simulink model "state_space_all_reduce_uio"  (R2018a)
settings: Solver=FixedStepAuto  StartTime=0.0  StopTime=3  FixedStep=tm  MaxStep=1e-4  RelTol=1e-5  AbsTol=1e-5
InitFcn:
  | SimulinkInit_linea_transmision
values from neighbouring files (symbols this model uses):
  b = 4.91    [SimulinkInit_linea_transmision.m]
  C = 1    [SimulinkInit_linea_transmision.m]
  C1 = 22e-6    (= 2.2e-05)    [SimulinkInit_linea_transmision.m]
  C2 = 22e-6    (= 2.2e-05)    [SimulinkInit_linea_transmision.m]
  C3 = 610e-6    (= 0.00061)    [SimulinkInit_linea_transmision.m]
  Cl = 20000e-6    (= 0.02)    [SimulinkInit_linea_transmision.m]
  Jd = 0.3    [SimulinkInit_linea_transmision.m]
  K = 25    [SimulinkInit_linea_transmision.m]    (also in uio_linear.m = K1+E*H)
  K1 = 9.66    [SimulinkInit_linea_transmision.m]    (also in uio_linear.m = K1')
  K11 = 0.8    [SimulinkInit_linea_transmision.m]
  K1d = 1.15    [SimulinkInit_linea_transmision.m]
  K2 = 6.97    [SimulinkInit_linea_transmision.m]
  K22 = 0.2    [SimulinkInit_linea_transmision.m]
  K2d = 1    [SimulinkInit_linea_transmision.m]
  K3 = 31.8    [SimulinkInit_linea_transmision.m]
  K33 = 0.23    [SimulinkInit_linea_transmision.m]
  K3d = 1    [SimulinkInit_linea_transmision.m]
  K4 = 15.1    [SimulinkInit_linea_transmision.m]
  Kd = 0.02    [SimulinkInit_linea_transmision.m]
  Kdc = 0.02    [SimulinkInit_linea_transmision.m]
  Kf = 1    [SimulinkInit_linea_transmision.m]
  Kh = 1.2    [SimulinkInit_linea_transmision.m]
  Ks = 21.5    [SimulinkInit_linea_transmision.m]
  Ksc = 3    [SimulinkInit_linea_transmision.m]
  Kv = 1    [SimulinkInit_linea_transmision.m]
  L = 5.2    [SimulinkInit_linea_transmision.m]
  L1 = 40e-3    (= 0.04)    [SimulinkInit_linea_transmision.m]
  L2 = 30e-3    (= 0.03)    [SimulinkInit_linea_transmision.m]
  L3 = 5e-3    (= 0.005)    [SimulinkInit_linea_transmision.m]
  L4 = 35e-6    (= 3.5e-05)    [SimulinkInit_linea_transmision.m]
  L5 = 22e-6    (= 2.2e-05)    [SimulinkInit_linea_transmision.m]
  L6 = 10e-6    (= 1e-05)    [SimulinkInit_linea_transmision.m]
  Pd = 0.1    [SimulinkInit_linea_transmision.m]
  R = 10    [SimulinkInit_linea_transmision.m]
  R1 = 0.1    [SimulinkInit_linea_transmision.m]
  R2 = 0.2    [SimulinkInit_linea_transmision.m]
  R3 = 1e-3    (= 0.001)    [SimulinkInit_linea_transmision.m]
  R4 = 0.005    [SimulinkInit_linea_transmision.m]
  R5 = 0.0012    [SimulinkInit_linea_transmision.m]
  R6 = 0.001    [SimulinkInit_linea_transmision.m]
  RL = 10    [SimulinkInit_linea_transmision.m]
  Sbin = 13.8    [SimulinkInit_linea_transmision.m]
  Svin = 2.91    [SimulinkInit_linea_transmision.m]
  T1 = 0.4    [SimulinkInit_linea_transmision.m]
  T2 = 1    [SimulinkInit_linea_transmision.m]
  T3 = 15    [SimulinkInit_linea_transmision.m]
  T4 = 2.5    [SimulinkInit_linea_transmision.m]
  Tao1d = 0.5    [SimulinkInit_linea_transmision.m]
  Tao2d = 0.125    [SimulinkInit_linea_transmision.m]
  Tcd = 0.2    [SimulinkInit_linea_transmision.m]
  Tcr = 0.01    [SimulinkInit_linea_transmision.m]
  Tf = 0.04    [SimulinkInit_linea_transmision.m]
  Tr = 950    [SimulinkInit_linea_transmision.m]
  Tt = 450    [SimulinkInit_linea_transmision.m]
  Ttd = 0.04    [SimulinkInit_linea_transmision.m]
  Tv = 0.05    [SimulinkInit_linea_transmision.m]
  V = 20    [SimulinkInit_linea_transmision.m]
  wref = 70000    [SimulinkInit_linea_transmision.m]
  X_acid = 1.2    [SimulinkInit_linea_transmision.m]
  X_meth = 0.35    [SimulinkInit_linea_transmision.m]
  Z = 3    [SimulinkInit_linea_transmision.m]
undefined symbols (not defined in the file or in its folder): Ad, ataque, Bd, c11, c12, c13, c14, C1o, c21, c22, c23, c24, C2o, c31, c32, c33, c34, C3o, c41, c42, c43, c44, C4o, Cd, F1, F2, F3, F4, H1, H2, H3, H4, K1U, K2U, K3U, K4U, T1s, T2s, T3s, T4s, T5s, tao1, tao2, taod, tm, uio1r, uio2r, uio3r, uio4r
libraries: neural x277, dsparch4 x4, powerlib_meascontrol x4, mpclib x1, simulink x1
(part 13 of 16)

== system state_space_all_reduce_uio/Function Fitting Neural Network3/Layer 2/Delays 1 ==
  "p{2}" : Inport  PortDimensions=30  SampleTime=4e-05
      mask Display: e = 0.06;c1 = [120 230 180]/255;c2 = ([120 230 180]+0)/(256+128);c3 = ([120 230 180]+128)/(256+128);patch([0 1 1 0],[0 0 1 1],c1);patch([0 1 1 1-e 1-e 0+e],[0 0 1 1-e 0+e 0+e],c2);patch([0 0 1 1-e 0+e 0+e],[0 1 1 1-e 1-e 0+e],c3);plot([0 1 1 0 0],[0 0 1 1 0]);
  mux : Mux  Inputs=1
      mask Display: e = 0.06;c1 = [120 150 230]/255;c2 = ([120 150 230]+0)/383;c3 = ([120 150 230]+128)/383;patch([0 1 1 0],[0 0 1 1],c1);patch([0 1 1 1-e 1-e 0+e],[0 0 1 1-e 0+e 0+e],c2);patch([0 0 1 1-e 0+e 0+e],[0 1 1 1-e 1-e 0+e],c3);plot([0 1 1 0 0],[0 0 1 1 0]);disp('Mux')
  "pd{2,1}" : Outport
      mask Display: e = 0.06;c1 = [120 230 180]/255;c2 = ([120 230 180]+0)/(256+128);c3 = ([120 230 180]+128)/(256+128);patch([0 1 1 0],[0 0 1 1],c1);patch([0 1 1 1-e 1-e 0+e],[0 0 1 1-e 0+e 0+e],c2);patch([0 0 1 1-e 0+e 0+e],[0 1 1 1-e 1-e 0+e],c3);plot([0 1 1 0 0],[0 0 1 1 0]);
  wires:
  "p{2}"/1 -> mux/1
  mux/1 -> "pd{2,1}"/1

== system state_space_all_reduce_uio/Function Fitting Neural Network3/Layer 2/LW{2,1} ==
  "ad{2,1}" : Inport  PortDimensions=30  SampleTime=4e-05
      mask Display: e = 0.06;c1 = [120 230 180]/255;c2 = ([120 230 180]+0)/(256+128);c3 = ([120 230 180]+128)/(256+128);patch([0 1 1 0],[0 0 1 1],c1);patch([0 1 1 1-e 1-e 0+e],[0 0 1 1-e 0+e 0+e],c2);patch([0 0 1 1-e 0+e 0+e],[0 1 1 1-e 1-e 0+e],c3);plot([0 1 1 0 0],[0 0 1 1 0]);
  "IW{2,1}(1,:)'" : Constant  Value=[-0.6108993563619720124080458845128305256366729736328125;-0.12377232021656990601510273108942783437669277191162109375;0.1986228164965912201811448767330148257315158843994140625;-0.2986234053889535999815052491612732410430908203125;-0.499479986781841578391549774096347391605377197265625;0.4244651480066325976991947754868306219577789306640625;-0.56892590557261402128830241053947247564792633056640625;-0.008160168266792812430399095546817989088594913482666015625;-0.03471042600284690582412849835236556828022003173828125;0.1662913602541268021095532958497642539441585540771484375;-0.51339807969661965802998793151346035301685333251953125;-0.11035191841669016177274187384682591073215007781982421875;0.1065034098801362905106770995189435780048370361328125;-0.387752517916231997929799035773612558841705322265625;0.25666787341159469360007960858638398349285125732421875;0.31597885591342012023829965983168222010135650634765625;-0.0106467373515204653811050405920468620024621486663818359375;-0.277670620246377064521681177211576141417026519775390625;0.024228256254273113079467094621577416546642780303955078125;0.019751607031808678105466725583028164692223072052001953125;-0.2018324091793771979386207249262952245771884918212890625;0.2218729906426324394175253473804332315921783447265625;0.3252039273491564852491819692659191787242889404296875;-0.274281505206600051405274598437245003879070281982421875;-0.149986905934014702612699920791783370077610015869140625;-0.229671358200306652275202168311807326972484588623046875;0.04070518967057305814716272607256541959941387176513671875;0.111095475677139010617366920996573753654956817626953125;-0.1194110113288310015544624320682487450540065765380859375;-0.00788339909671024151316398587141520692966878414154052734375]
      mask Display: e = 0.06;c1 = [120 150 230]/255;c2 = ([120 150 230]+0)/383;c3 = ([120 150 230]+128)/383;patch([0 1 1 0],[0 0 1 1],c1);patch([0 1 1 1-e 1-e 0+e],[0 0 1 1-e 0+e 0+e],c2);patch([0 0 1 1-e 0+e 0+e],[0 1 1 1-e 1-e 0+e],c3);plot([0 1 1 0 0],[0 0 1 1 0]);disp('weights');
  "IW{2,1}(10,:)'" : Constant  Value=[0.29635779515491955660166922825737856328487396240234375;0.2034166761778584409103842745025758631527423858642578125;-0.0023683642057664463891064610123748934711329638957977294921875;0.22124729721162073037277195908245630562305450439453125;0.3369155378131185596402019655215553939342498779296875;0.1500263956989058289348548669295269064605236053466796875;-0.2497175765352100118565914499413338489830493927001953125;-0.10301693128462863224825696306652389466762542724609375;-0.01099510239059186579579918685567463398911058902740478515625;0.115527621161523430526330002976465038955211639404296875;0.0692645313952721386474564724267111159861087799072265625;0.0119651086510804242901695459977418067865073680877685546875;0.290075191506396434792947047753841616213321685791015625;0.2032135105828389021187518892475054599344730377197265625;-0.0211155493846143203773291219249585992656648159027099609375;0.1060308181848053921125796250635175965726375579833984375;-0.1181015704355025397465084324721829034388065338134765625;0.45860412450985454935192819903022609651088714599609375;-0.20160056133213621887279032307560555636882781982421875;-0.1021768772968167648951265391588094644248485565185546875;-0.463237381515118007424547386108315549790859222412109375;-0.09568885509427126068171531869666068814694881439208984375;0.052744303583831746162768894237160566262900829315185546875;0.0475424460660857917115862392165581695735454559326171875;-0.0035101213614650308113274146393223418272100389003753662109375;-0.25541990716382245718563126501976512372493743896484375;0.528868712182579248093361456994898617267608642578125;-0.295106782712837356630330987172783352434635162353515625;-0.082279435194425432076315019003232009708881378173828125;0.07298068872108949556309909212359343655407428741455078125]
      mask Display: e = 0.06;c1 = [120 150 230]/255;c2 = ([120 150 230]+0)/383;c3 = ([120 150 230]+128)/383;patch([0 1 1 0],[0 0 1 1],c1);patch([0 1 1 1-e 1-e 0+e],[0 0 1 1-e 0+e 0+e],c2);patch([0 0 1 1-e 0+e 0+e],[0 1 1 1-e 1-e 0+e],c3);plot([0 1 1 0 0],[0 0 1 1 0]);disp('weights');
  "IW{2,1}(2,:)'" : Constant  Value=[0.09708916544488814526214781608359771780669689178466796875;0.2255772120654304380149568487468059174716472625732421875;0.003702961884490557457894066573089730809442698955535888671875;0.029624972225403896353146393494171206839382648468017578125;-0.1954796502596932439299592942916206084191799163818359375;-0.59940544466154144220837451939587481319904327392578125;0.260557299906677253265030458351247943937778472900390625;-0.63305372508061619196695346545311622321605682373046875;-0.295649046001520476867341358229168690741062164306640625;0.04053401399485075107254061776984599418938159942626953125;-0.046834290540188054652315230441672611050307750701904296875;0.08317365441290917871253185467139701358973979949951171875;0.17331529140582990766716875441488809883594512939453125;0.0275578103417470389457921697839992702938616275787353515625;0.2018023672489276665320545589565881527960300445556640625;0.06743810023460482250268199777565314434468746185302734375;-0.180275428148382765858315224249963648617267608642578125;-0.2579369278587984037898195310845039784908294677734375;-0.0921851184035180903908468508234363980591297149658203125;0.061569880123684785078186365581132122315466403961181640625;0.314599908239820258426533428064431063830852508544921875;-0.0131290228955344666361693128919796436093747615814208984375;0.033185419198564942988571857540591736324131488800048828125;-0.00933833744509623801810516141586049343459308147430419921875;-0.1033221182311379326979050574664142914116382598876953125;-0.1921781391607385869324531313395709730684757232666015625;0.055416200609459266568368462912985705770552158355712890625;-0.1488744040050123673690762871046899817883968353271484375;0.2094008490666214028497194021838367916643619537353515625;0.046990537131259495218227328905413742177188396453857421875]
      mask Display: e = 0.06;c1 = [120 150 230]/255;c2 = ([120 150 230]+0)/383;c3 = ([120 150 230]+128)/383;patch([0 1 1 0],[0 0 1 1],c1);patch([0 1 1 1-e 1-e 0+e],[0 0 1 1-e 0+e 0+e],c2);patch([0 0 1 1-e 0+e 0+e],[0 1 1 1-e 1-e 0+e],c3);plot([0 1 1 0 0],[0 0 1 1 0]);disp('weights');
  "IW{2,1}(3,:)'" : Constant  Value=[0.12460931784415903156304494814321515150368213653564453125;-0.35778269794602979292363897911855019629001617431640625;0.023278058036042138800869594206233159638941287994384765625;-0.268905202381384544896292254634317941963672637939453125;0.2125526564810290286455796149311936460435390472412109375;-0.332587259490805531303436737289302982389926910400390625;-0.1870172122518136970104052352326107211410999298095703125;-0.294072954416423726353713163916836492717266082763671875;0.0670400945985989149544792553570005111396312713623046875;0.0215328682295782801447980858711161999963223934173583984375;0.00893792162565088151027214991017899592407047748565673828125;-0.09649036626923256088073088676537736319005489349365234375;0.052689337275451102182710627630513045005500316619873046875;-0.21281430046342431072758927257382310926914215087890625;0.0208968278071027489806166244079577154479920864105224609375;0.0667961657798825658716168618411757051944732666015625;-0.00069132157059649773471476930097878721426241099834442138671875;-0.050070962703474962418592753010671003721654415130615234375;-0.08289314228870196810117221275504562072455883026123046875;0.037986939224426252703636919250129722058773040771484375;0.181202224291058422434019803404225967824459075927734375;0.274506776572543020886740805508452467620372772216796875;0.02977815686653696725105788800647133029997348785400390625;0.2139927463900734572188611082310671918094158172607421875;-0.162725233885205933237472208929830230772495269775390625;-0.019048537270349642780420396093177259899675846099853515625;0.0786097109228997836805064025611500255763530731201171875;-0.205967836298671047590147509254165925085544586181640625;0.479129205120557177810525217864778824150562286376953125;-0.2132697439127679006620752488743164576590061187744140625]
      mask Display: e = 0.06;c1 = [120 150 230]/255;c2 = ([120 150 230]+0)/383;c3 = ([120 150 230]+128)/383;patch([0 1 1 0],[0 0 1 1],c1);patch([0 1 1 1-e 1-e 0+e],[0 0 1 1-e 0+e 0+e],c2);patch([0 0 1 1-e 0+e 0+e],[0 1 1 1-e 1-e 0+e],c3);plot([0 1 1 0 0],[0 0 1 1 0]);disp('weights');
  "IW{2,1}(4,:)'" : Constant  Value=[-0.19633352528214498278202881920151412487030029296875;-0.121800271312692609537720045409514568746089935302734375;-0.0182132757588536510484633623718764283694326877593994140625;0.04471817409413435251419599580913200043141841888427734375;-0.0108854916126952215582601724008782184682786464691162109375;0.1332237321224387371909614330434123985469341278076171875;-0.146363427813941460176039299767580814659595489501953125;-0.0711709499843555526421567947181756608188152313232421875;0.25548925411243594840726700567756779491901397705078125;-0.059906029830572193883853060469846241176128387451171875;-0.1773225990205870850058289533990318886935710906982421875;-0.128281540302648655593742432756698690354824066162109375;0.039306928108965459578438839116643066518008708953857421875;-0.1122515827125971643596358262584544718265533447265625;-0.221202886936299247810921997370314784348011016845703125;0.006098252527073856101014204256216544308699667453765869140625;0.1596102041277631389259994421081501059234142303466796875;-0.1825895981040427107355839098090655170381069183349609375;0.11478182843430244364224535047469544224441051483154296875;0.0232732308372753417258227415231885970570147037506103515625;-0.3765874921128109509282921862904913723468780517578125;-0.0699864919821701347846243379535735584795475006103515625;-0.00106709298812400553251034107660188965382985770702362060546875;0.160946111283145787407278248792863450944423675537109375;0.153627959179783724064094485584064386785030364990234375;-0.01129040371139962591062744223791014519520103931427001953125;-0.1923537583599702893710770013058208860456943511962890625;-0.146999298339756057085736529188579879701137542724609375;-0.459863329862106595680160125994007103145122528076171875;-0.1125495018655740253610275658502359874546527862548828125]
      mask Display: e = 0.06;c1 = [120 150 230]/255;c2 = ([120 150 230]+0)/383;c3 = ([120 150 230]+128)/383;patch([0 1 1 0],[0 0 1 1],c1);patch([0 1 1 1-e 1-e 0+e],[0 0 1 1-e 0+e 0+e],c2);patch([0 0 1 1-e 0+e 0+e],[0 1 1 1-e 1-e 0+e],c3);plot([0 1 1 0 0],[0 0 1 1 0]);disp('weights');
  "IW{2,1}(5,:)'" : Constant  Value=[-0.341502604101319884311038777013891376554965972900390625;0.038566451327512678293185643951801466755568981170654296875;-0.1395052210143926940677516768118948675692081451416015625;0.10063509544883060542463937281354446895420551300048828125;0.1815214851574560028790727983505348674952983856201171875;-0.434218928709956430989080899962573312222957611083984375;0.408667171366868309245745649604941718280315399169921875;0.385137624400757994092003855257644318044185638427734375;-0.35508535953012343444612497478374280035495758056640625;0.395894896479553282109264955579419620335102081298828125;-0.441418591976789453923402106738649308681488037109375;0.468883832187682703107611814630217850208282470703125;0.452535260372043612875359031022526323795318603515625;-0.435690587373383897418221977204666472971439361572265625;-0.14185885407803755509092979991692118346691131591796875;0.272747534495510091101522220924380235373973846435546875;0.04098815291252873305172244045024854131042957305908203125;-0.3307976810063457673294351479853503406047821044921875;0.2101715684222978108852686318641644902527332305908203125;-0.1539716328844354109595116142372717149555683135986328125;-0.272987765307725449570597220372292213141918182373046875;0.305095574115205658838334557003690861165523529052734375;-0.04287979135288509657808475594720221124589443206787109375;-0.41147834133321092853208256201469339430332183837890625;0.53712368878818439466016343430965207517147064208984375;0.416191517197288474161354088209918700158596038818359375;0.04749985538923630346008764036014326848089694976806640625;-0.1798369007383437689906457990218768827617168426513671875;0.01525251243919280297323126660558045841753482818603515625;-0.54013565597617951841158401293796487152576446533203125]
      mask Display: e = 0.06;c1 = [120 150 230]/255;c2 = ([120 150 230]+0)/383;c3 = ([120 150 230]+128)/383;patch([0 1 1 0],[0 0 1 1],c1);patch([0 1 1 1-e 1-e 0+e],[0 0 1 1-e 0+e 0+e],c2);patch([0 0 1 1-e 0+e 0+e],[0 1 1 1-e 1-e 0+e],c3);plot([0 1 1 0 0],[0 0 1 1 0]);disp('weights');
  "IW{2,1}(6,:)'" : Constant  Value=[0.49925490638036185142567546790814958512783050537109375;0.12402283349013844271357953630285919643938541412353515625;0.07420110878195196324469407045398838818073272705078125;-0.268528915716013505399217820013291202485561370849609375;0.462956992662289235074268844982725568115711212158203125;-0.007515270830356904872837642272997982217930257320404052734375;-0.481571654503173796069148693277384154498577117919921875;-0.08387177086194898267823560900069423951208591461181640625;-0.52940697956280036162723945381003431975841522216796875;0.323217987371589021705631239456124603748321533203125;0.1568066838196668921767695792368613183498382568359375;0.40583622791357065739958898120676167309284210205078125;0.08930773221745569312446377807646058499813079833984375;-0.3258180832558463801973402951261959969997406005859375;0.1402346353061940387174644229162367992103099822998046875;-0.202497063814745581478149460963322781026363372802734375;-0.030890754278159980594775646522975875996053218841552734375;0.1144440458135578264631249112426303327083587646484375;-0.52332038790228008195981601602397859096527099609375;0.0205082634168946252584131428875480196438729763031005859375;-0.140059324007881846885226195809082128107547760009765625;0.0227385631742271603072946817292177001945674419403076171875;0.04104951059130988733070211083031608723104000091552734375;-0.44803892833890424096665583419962786138057708740234375;-0.455430901449709046868719042322481982409954071044921875;0.34017445856057137998362804864882491528987884521484375;-0.52777334503266215559591501005343161523342132568359375;0.61711177965770447340076998443691991269588470458984375;-0.1172188000697740317690431766095571219921112060546875;0.049266357298894093708074848336764262057840824127197265625]
      mask Display: e = 0.06;c1 = [120 150 230]/255;c2 = ([120 150 230]+0)/383;c3 = ([120 150 230]+128)/383;patch([0 1 1 0],[0 0 1 1],c1);patch([0 1 1 1-e 1-e 0+e],[0 0 1 1-e 0+e 0+e],c2);patch([0 0 1 1-e 0+e 0+e],[0 1 1 1-e 1-e 0+e],c3);plot([0 1 1 0 0],[0 0 1 1 0]);disp('weights');
  "IW{2,1}(7,:)'" : Constant  Value=[0.036708599756844435824110206567638670094311237335205078125;0.1096854095616091318010631994184223003685474395751953125;-0.022078643810732691277198824764127493835985660552978515625;0.61378380423222866912880135714658536016941070556640625;0.21004296218785778460613755669328384101390838623046875;-0.51994852170594063611730462071136571466922760009765625;-0.57842560919090224569316660563345067203044891357421875;0.097160600096388438640104823207366280257701873779296875;-0.37978985583719782059830549769685603678226470947265625;-0.07765784517062475356130590853354078717529773712158203125;-0.20417782875814849408158124788315035402774810791015625;-0.1448559489658842458492671312342281453311443328857421875;-0.1997818239064153844619653455083607695996761322021484375;-0.50620673707847718691965610560146160423755645751953125;-0.2243158369550604935849236198919243179261684417724609375;-0.06966453684462425854917455581016838550567626953125;0.299991235207171025312078427305095829069614410400390625;-0.1099435947310898609163842820635181851685047149658203125;0.1624020068420821971688638996056397445499897003173828125;-0.054784390240681206385442436612720484845340251922607421875;0.43531344416034845057339452978339977562427520751953125;0.2052756780230019229005478109684190712869167327880859375;-0.049654717239222601055104178158217109739780426025390625;0.07186210672408070709860083979947376064956188201904296875;0.429542962623020441181864725876948796212673187255859375;0.1707548603417280153049517821273184381425380706787109375;-0.46502172346302972361087313402094878256320953369140625;0.064153631383797760090459405546425841748714447021484375;-0.20833364336469906152871089943801052868366241455078125;-0.1460654280552280692706546005865675397217273712158203125]
      mask Display: e = 0.06;c1 = [120 150 230]/255;c2 = ([120 150 230]+0)/383;c3 = ([120 150 230]+128)/383;patch([0 1 1 0],[0 0 1 1],c1);patch([0 1 1 1-e 1-e 0+e],[0 0 1 1-e 0+e 0+e],c2);patch([0 0 1 1-e 0+e 0+e],[0 1 1 1-e 1-e 0+e],c3);plot([0 1 1 0 0],[0 0 1 1 0]);disp('weights');
  "IW{2,1}(8,:)'" : Constant  Value=[0.36685370791122784428495151587412692606449127197265625;-0.0395954107167282021162435512451338581740856170654296875;0.00752315304133420285903621760326132061891257762908935546875;-0.2011594708128000286162517795673920772969722747802734375;0.1509921968677504777733844321119249798357486724853515625;0.43163337538544277460772491394891403615474700927734375;-0.05987998631625758572116779987482004798948764801025390625;-0.09427629929722335100361618742681457661092281341552734375;-0.0359046790899595347212880369625054299831390380859375;0.27321007671768515745469585453975014388561248779296875;0.430747708124629813397632460691966116428375244140625;-0.12489902345915837589274133279104717075824737548828125;-0.19101566414585746667142984733800403773784637451171875;0.45344389015841735091072450813953764736652374267578125;0.325825664675891302213273093002499081194400787353515625;0.45359923507634880568417656832025386393070220947265625;-0.093285872675504422080194899535854347050189971923828125;-0.46228372500059389249571495383861474692821502685546875;-0.1755167482854316507445702200129744596779346466064453125;-0.12302806366879241728451432891233707778155803680419921875;-0.3352889352977099779451464200974442064762115478515625;0.13946840122542358830770581334945745766162872314453125;0.1720945696979952199701102699691546149551868438720703125;-0.27490795331073225593598863270017318427562713623046875;0.048575503819257119519914311922548222355544567108154296875;-0.425562630221491822180013286924804560840129852294921875;-0.1473218360246301428251314291628659702837467193603515625;-0.369330926269416714990967420817469246685504913330078125;0.03615173273082054883342806306245620362460613250732421875;-0.0156354739191119258834294925009089638479053974151611328125]
      mask Display: e = 0.06;c1 = [120 150 230]/255;c2 = ([120 150 230]+0)/383;c3 = ([120 150 230]+128)/383;patch([0 1 1 0],[0 0 1 1],c1);patch([0 1 1 1-e 1-e 0+e],[0 0 1 1-e 0+e 0+e],c2);patch([0 0 1 1-e 0+e 0+e],[0 1 1 1-e 1-e 0+e],c3);plot([0 1 1 0 0],[0 0 1 1 0]);disp('weights');
  "IW{2,1}(9,:)'" : Constant  Value=[-0.48325833622205749406930408440530300140380859375;0.57649331399421155364137803189805708825588226318359375;0.11458788256533876392939674815352191217243671417236328125;-0.1534774723912077643017681793935480527579784393310546875;0.402973241251314562294538745845784433186054229736328125;0.135367724806911005064335995484725572168827056884765625;-0.317286799267680663660939899273216724395751953125;0.360933051219507750051462835472193546593189239501953125;0.02686544720392568252886889013097970746457576751708984375;0.03190093588507403321585798039450310170650482177734375;0.24413470064272912996017339537502266466617584228515625;0.165929246360893511980094672253471799194812774658203125;-0.28656476216798321132728233351372182369232177734375;0.09208865865231834202386806964568677358329296112060546875;0.376343732856873225411931116468622349202632904052734375;-0.1880254341477767265899956328212283551692962646484375;0.0167034276740541977324117084435783908702433109283447265625;0.4015984837593713496772807047818787395954132080078125;-0.269968765506449492885820973242516629397869110107421875;-0.0220835346860907520694095040880711167119443416595458984375;-0.6551298345222693608747022153693251311779022216796875;0.1822989509266637886408801705329096876084804534912109375;-0.16428222144759152545390179511741735041141510009765625;-0.1600282180942602383577622049415367655456066131591796875;-0.64081508504144124582779795673559419810771942138671875;-0.342499255805971458688219399846275337040424346923828125;0.61734497873460802974676653320784680545330047607421875;0.132281991580877555936268663572263903915882110595703125;0.136239989197204647286554290985804982483386993408203125;0.30769750869183465358247531185043044388294219970703125]
      mask Display: e = 0.06;c1 = [120 150 230]/255;c2 = ([120 150 230]+0)/383;c3 = ([120 150 230]+128)/383;patch([0 1 1 0],[0 0 1 1],c1);patch([0 1 1 1-e 1-e 0+e],[0 0 1 1-e 0+e 0+e],c2);patch([0 0 1 1-e 0+e 0+e],[0 1 1 1-e 1-e 0+e],c3);plot([0 1 1 0 0],[0 0 1 1 0]);disp('weights');
  Mux : Mux  Inputs=10
      mask Display: e = 0.06;c1 = [120 150 230]/255;c2 = ([120 150 230]+0)/383;c3 = ([120 150 230]+128)/383;patch([0 1 1 0],[0 0 1 1],c1);patch([0 1 1 1-e 1-e 0+e],[0 0 1 1-e 0+e 0+e],c2);patch([0 0 1 1-e 0+e 0+e],[0 1 1 1-e 1-e 0+e],c3);plot([0 1 1 0 0],[0 0 1 1 0]);disp('Mux');
  dotprod{1..10} (10 alike) : neural/Weight Functions/dotprod
  "lz{2,1}" : Outport
      mask Display: e = 0.06;c1 = [120 230 180]/255;c2 = ([120 230 180]+0)/(256+128);c3 = ([120 230 180]+128)/(256+128);patch([0 1 1 0],[0 0 1 1],c1);patch([0 1 1 1-e 1-e 0+e],[0 0 1 1-e 0+e 0+e],c2);patch([0 0 1 1-e 0+e 0+e],[0 1 1 1-e 1-e 0+e],c3);plot([0 1 1 0 0],[0 0 1 1 0]);
  wires:
  "IW{2,1}(1,:)'"/1 -> dotprod1/1
  "ad{2,1}"/1 -> dotprod1/2, dotprod2/2, dotprod3/2, dotprod4/2, dotprod5/2, dotprod6/2, dotprod7/2, dotprod8/2, dotprod9/2, dotprod10/2
  dotprod1/1 -> Mux/1
  "IW{2,1}(2,:)'"/1 -> dotprod2/1
  dotprod2/1 -> Mux/2
  "IW{2,1}(3,:)'"/1 -> dotprod3/1
  dotprod3/1 -> Mux/3
  "IW{2,1}(4,:)'"/1 -> dotprod4/1
  dotprod4/1 -> Mux/4
  "IW{2,1}(5,:)'"/1 -> dotprod5/1
  dotprod5/1 -> Mux/5
  "IW{2,1}(6,:)'"/1 -> dotprod6/1
  dotprod6/1 -> Mux/6
  "IW{2,1}(7,:)'"/1 -> dotprod7/1
  dotprod7/1 -> Mux/7
  "IW{2,1}(8,:)'"/1 -> dotprod8/1
  dotprod8/1 -> Mux/8
  "IW{2,1}(9,:)'"/1 -> dotprod9/1
  dotprod9/1 -> Mux/9
  "IW{2,1}(10,:)'"/1 -> dotprod10/1
  dotprod10/1 -> Mux/10
  Mux/1 -> "lz{2,1}"/1

== system state_space_all_reduce_uio/Function Fitting Neural Network3/Layer 3/Delays 1 ==
  "p{3}" : Inport  PortDimensions=10  SampleTime=4e-05
      mask Display: e = 0.06;c1 = [120 230 180]/255;c2 = ([120 230 180]+0)/(256+128);c3 = ([120 230 180]+128)/(256+128);patch([0 1 1 0],[0 0 1 1],c1);patch([0 1 1 1-e 1-e 0+e],[0 0 1 1-e 0+e 0+e],c2);patch([0 0 1 1-e 0+e 0+e],[0 1 1 1-e 1-e 0+e],c3);plot([0 1 1 0 0],[0 0 1 1 0]);
  mux : Mux  Inputs=1
      mask Display: e = 0.06;c1 = [120 150 230]/255;c2 = ([120 150 230]+0)/383;c3 = ([120 150 230]+128)/383;patch([0 1 1 0],[0 0 1 1],c1);patch([0 1 1 1-e 1-e 0+e],[0 0 1 1-e 0+e 0+e],c2);patch([0 0 1 1-e 0+e 0+e],[0 1 1 1-e 1-e 0+e],c3);plot([0 1 1 0 0],[0 0 1 1 0]);disp('Mux')
  "pd{3,2}" : Outport
      mask Display: e = 0.06;c1 = [120 230 180]/255;c2 = ([120 230 180]+0)/(256+128);c3 = ([120 230 180]+128)/(256+128);patch([0 1 1 0],[0 0 1 1],c1);patch([0 1 1 1-e 1-e 0+e],[0 0 1 1-e 0+e 0+e],c2);patch([0 0 1 1-e 0+e 0+e],[0 1 1 1-e 1-e 0+e],c3);plot([0 1 1 0 0],[0 0 1 1 0]);
  wires:
  "p{3}"/1 -> mux/1
  mux/1 -> "pd{3,2}"/1

== system state_space_all_reduce_uio/Function Fitting Neural Network3/Layer 3/LW{3,2} ==
  "ad{3,2}" : Inport  PortDimensions=10  SampleTime=4e-05
      mask Display: e = 0.06;c1 = [120 230 180]/255;c2 = ([120 230 180]+0)/(256+128);c3 = ([120 230 180]+128)/(256+128);patch([0 1 1 0],[0 0 1 1],c1);patch([0 1 1 1-e 1-e 0+e],[0 0 1 1-e 0+e 0+e],c2);patch([0 0 1 1-e 0+e 0+e],[0 1 1 1-e 1-e 0+e],c3);plot([0 1 1 0 0],[0 0 1 1 0]);
  "IW{3,2}(1,:)'" : Constant  Value=[0.274627997814195057291186685688444413244724273681640625;-0.474180215990095466072062890816596336662769317626953125;0.2603401288970326188376702702953480184078216552734375;0.8699100649256978901036063689389266073703765869140625;0.039836816239801127459418950138569925911724567413330078125;-0.53532080456377151289615312634850852191448211669921875;-0.95878607545585758931139253036235459148883819580078125;-0.039847664109300899581977972729873727075755596160888671875;0.10550380963504864262336724323176895268261432647705078125;-0.83915160663412546870887354089063592255115509033203125]
      mask Display: e = 0.06;c1 = [120 150 230]/255;c2 = ([120 150 230]+0)/383;c3 = ([120 150 230]+128)/383;patch([0 1 1 0],[0 0 1 1],c1);patch([0 1 1 1-e 1-e 0+e],[0 0 1 1-e 0+e 0+e],c2);patch([0 0 1 1-e 0+e 0+e],[0 1 1 1-e 1-e 0+e],c3);plot([0 1 1 0 0],[0 0 1 1 0]);disp('weights');
  "IW{3,2}(10,:)'" : Constant  Value=[-0.65551827401669993111710255107027478516101837158203125;0.0808923682628386597759373444205266423523426055908203125;-0.339434282337944315255384708507335744798183441162109375;-0.5614548586125198692542426215368323028087615966796875;-0.0238827821795674598293057755427071242593228816986083984375;-0.71962962389343820834852749612764455378055572509765625;-0.73782026776228681885783089455799199640750885009765625;-0.51125256196273005659946875312016345560550689697265625;-0.8536722189307870412022793971118517220020294189453125;0.016210077342749047712988641478659701533615589141845703125]
      mask Display: e = 0.06;c1 = [120 150 230]/255;c2 = ([120 150 230]+0)/383;c3 = ([120 150 230]+128)/383;patch([0 1 1 0],[0 0 1 1],c1);patch([0 1 1 1-e 1-e 0+e],[0 0 1 1-e 0+e 0+e],c2);patch([0 0 1 1-e 0+e 0+e],[0 1 1 1-e 1-e 0+e],c3);plot([0 1 1 0 0],[0 0 1 1 0]);disp('weights');
  "IW{3,2}(2,:)'" : Constant  Value=[-0.1341001663969128843145739438114105723798274993896484375;-1.119503785645471705123554784222505986690521240234375;0.326665273659767496639005912584252655506134033203125;0.6099654547035437968105497930082492530345916748046875;0.54728565185062338915855661980458535254001617431640625;-0.42152024985953240321379098531906493008136749267578125;0.44240936354143711728426069385022856295108795166015625;0.13520406605259005505814684511278755962848663330078125;0.60258588542572721902246257741353474557399749755859375;0.2326482944973339572758419535603024996817111968994140625]
      mask Display: e = 0.06;c1 = [120 150 230]/255;c2 = ([120 150 230]+0)/383;c3 = ([120 150 230]+128)/383;patch([0 1 1 0],[0 0 1 1],c1);patch([0 1 1 1-e 1-e 0+e],[0 0 1 1-e 0+e 0+e],c2);patch([0 0 1 1-e 0+e 0+e],[0 1 1 1-e 1-e 0+e],c3);plot([0 1 1 0 0],[0 0 1 1 0]);disp('weights');
  "IW{3,2}(3,:)'" : Constant  Value=[-0.371320237214100734579602658413932658731937408447265625;-0.89015330485143717709206612198613584041595458984375;-0.66449888741414497861370591635932214558124542236328125;-0.09636728243575416741339978443647851236164569854736328125;0.1220790936496769785168936550689977593719959259033203125;-0.1949565527260398167808119751498452387750148773193359375;-0.307053844965301137026614242131472565233707427978515625;-0.26662797554856509929521735102753154933452606201171875;-0.346555985614589057153267503963434137403964996337890625;0.230656408670605106436823916737921535968780517578125]
      mask Display: e = 0.06;c1 = [120 150 230]/255;c2 = ([120 150 230]+0)/383;c3 = ([120 150 230]+128)/383;patch([0 1 1 0],[0 0 1 1],c1);patch([0 1 1 1-e 1-e 0+e],[0 0 1 1-e 0+e 0+e],c2);patch([0 0 1 1-e 0+e 0+e],[0 1 1 1-e 1-e 0+e],c3);plot([0 1 1 0 0],[0 0 1 1 0]);disp('weights');
  "IW{3,2}(4,:)'" : Constant  Value=[-0.536244840634006347812601234181784093379974365234375;1.0737886042126962848897164803929626941680908203125;0.153908594350457728072711915956460870802402496337890625;0.267898151989196808830939744439092464745044708251953125;-0.99856560645589353963913481493364088237285614013671875;0.5389646684660143183265290645067580044269561767578125;0.1345200533332061854085992536056437529623508453369140625;-0.35532831099991113443792301040957681834697723388671875;-0.45041658594143962890399279785924591124057769775390625;-0.144701706081101721945714189132559113204479217529296875]
      mask Display: e = 0.06;c1 = [120 150 230]/255;c2 = ([120 150 230]+0)/383;c3 = ([120 150 230]+128)/383;patch([0 1 1 0],[0 0 1 1],c1);patch([0 1 1 1-e 1-e 0+e],[0 0 1 1-e 0+e 0+e],c2);patch([0 0 1 1-e 0+e 0+e],[0 1 1 1-e 1-e 0+e],c3);plot([0 1 1 0 0],[0 0 1 1 0]);disp('weights');
  "IW{3,2}(5,:)'" : Constant  Value=[0.6805868734006172982020643758005462586879730224609375;-0.3175490031171042115687441764748655259609222412109375;0.691691552356882510821378673426806926727294921875;0.2408526014150360328169853119106846861541271209716796875;-0.421923267204521390549842863038065843284130096435546875;-0.226139024500568719400206418868037872016429901123046875;0.823042895664465756766503545804880559444427490234375;0.60223082968826113781091180499061010777950286865234375;1.0086064178572173855030769118457101285457611083984375;0.060606053778316404390125171630643308162689208984375]
      mask Display: e = 0.06;c1 = [120 150 230]/255;c2 = ([120 150 230]+0)/383;c3 = ([120 150 230]+128)/383;patch([0 1 1 0],[0 0 1 1],c1);patch([0 1 1 1-e 1-e 0+e],[0 0 1 1-e 0+e 0+e],c2);patch([0 0 1 1-e 0+e 0+e],[0 1 1 1-e 1-e 0+e],c3);plot([0 1 1 0 0],[0 0 1 1 0]);disp('weights');
  "IW{3,2}(6,:)'" : Constant  Value=[0.8930968866877992962116650232928805053234100341796875;0.083736672909214104887354324091575108468532562255859375;0.7109637846387346638010740207391791045665740966796875;-0.37678184905507283719572342306491918861865997314453125;0.450137327733081626934819041707669384777545928955078125;-0.44785932090979574393685425093281082808971405029296875;0.464406294259891161413378313227440230548381805419921875;-0.11878211325429270661668823549916851334273815155029296875;0.006428457557057977271586235445965940016321837902069091796875;-0.75851347489151110803362598744570277631282806396484375]
      mask Display: e = 0.06;c1 = [120 150 230]/255;c2 = ([120 150 230]+0)/383;c3 = ([120 150 230]+128)/383;patch([0 1 1 0],[0 0 1 1],c1);patch([0 1 1 1-e 1-e 0+e],[0 0 1 1-e 0+e 0+e],c2);patch([0 0 1 1-e 0+e 0+e],[0 1 1 1-e 1-e 0+e],c3);plot([0 1 1 0 0],[0 0 1 1 0]);disp('weights');
  "IW{3,2}(7,:)'" : Constant  Value=[-0.6990696598700287811567477547214366495609283447265625;0.864164235340528552598016176489181816577911376953125;0.12496553734751376929512645119757507927715778350830078125;0.5771548115341686990831249204347841441631317138671875;0.03814162689538504180664091336439014412462711334228515625;-0.96400013729871314449582087036105804145336151123046875;0.61642513594585046643459236292983405292034149169921875;0.798589904338348421930504628107883036136627197265625;-0.4572775432386502192372290664934553205966949462890625;-0.400377693403756451662189874696196056902408599853515625]
      mask Display: e = 0.06;c1 = [120 150 230]/255;c2 = ([120 150 230]+0)/383;c3 = ([120 150 230]+128)/383;patch([0 1 1 0],[0 0 1 1],c1);patch([0 1 1 1-e 1-e 0+e],[0 0 1 1-e 0+e 0+e],c2);patch([0 0 1 1-e 0+e 0+e],[0 1 1 1-e 1-e 0+e],c3);plot([0 1 1 0 0],[0 0 1 1 0]);disp('weights');
  "IW{3,2}(8,:)'" : Constant  Value=[0.8307707717163628213796755517250858247280120849609375;0.066721617497039253930068980480427853763103485107421875;-0.78624522819443942722728024818934500217437744140625;0.07483548304229341308069223259735736064612865447998046875;-0.9649915265665891528357178685837425291538238525390625;-0.492886857767258435014667838913737796247005462646484375;-0.2136935428089402344564717850516899488866329193115234375;0.19646378943504572145428710427950136363506317138671875;0.390122346073913883746087094550603069365024566650390625;0.68059632724051499774731155412155203521251678466796875]
      mask Display: e = 0.06;c1 = [120 150 230]/255;c2 = ([120 150 230]+0)/383;c3 = ([120 150 230]+128)/383;patch([0 1 1 0],[0 0 1 1],c1);patch([0 1 1 1-e 1-e 0+e],[0 0 1 1-e 0+e 0+e],c2);patch([0 0 1 1-e 0+e 0+e],[0 1 1 1-e 1-e 0+e],c3);plot([0 1 1 0 0],[0 0 1 1 0]);disp('weights');
  "IW{3,2}(9,:)'" : Constant  Value=[-0.31801254154562352827184668058180250227451324462890625;-0.8944843465739136245673535086098127067089080810546875;0.008128930529336296506581760468179709278047084808349609375;0.09565144225893219831480251968969241715967655181884765625;0.267912282400417922634261458370019681751728057861328125;-0.60627655979721861712050667847506701946258544921875;0.57371306159595547580209995430777780711650848388671875;-0.296012641519426134006920392494066618382930755615234375;0.54141925677320357213062607115716673433780670166015625;0.259031680873608838311383806285448372364044189453125]
      mask Display: e = 0.06;c1 = [120 150 230]/255;c2 = ([120 150 230]+0)/383;c3 = ([120 150 230]+128)/383;patch([0 1 1 0],[0 0 1 1],c1);patch([0 1 1 1-e 1-e 0+e],[0 0 1 1-e 0+e 0+e],c2);patch([0 0 1 1-e 0+e 0+e],[0 1 1 1-e 1-e 0+e],c3);plot([0 1 1 0 0],[0 0 1 1 0]);disp('weights');
  Mux : Mux  Inputs=10
      mask Display: e = 0.06;c1 = [120 150 230]/255;c2 = ([120 150 230]+0)/383;c3 = ([120 150 230]+128)/383;patch([0 1 1 0],[0 0 1 1],c1);patch([0 1 1 1-e 1-e 0+e],[0 0 1 1-e 0+e 0+e],c2);patch([0 0 1 1-e 0+e 0+e],[0 1 1 1-e 1-e 0+e],c3);plot([0 1 1 0 0],[0 0 1 1 0]);disp('Mux');
  dotprod{1..10} (10 alike) : neural/Weight Functions/dotprod
  "lz{3,2}" : Outport
      mask Display: e = 0.06;c1 = [120 230 180]/255;c2 = ([120 230 180]+0)/(256+128);c3 = ([120 230 180]+128)/(256+128);patch([0 1 1 0],[0 0 1 1],c1);patch([0 1 1 1-e 1-e 0+e],[0 0 1 1-e 0+e 0+e],c2);patch([0 0 1 1-e 0+e 0+e],[0 1 1 1-e 1-e 0+e],c3);plot([0 1 1 0 0],[0 0 1 1 0]);
  wires:
  "IW{3,2}(1,:)'"/1 -> dotprod1/1
  "ad{3,2}"/1 -> dotprod1/2, dotprod2/2, dotprod3/2, dotprod4/2, dotprod5/2, dotprod6/2, dotprod7/2, dotprod8/2, dotprod9/2, dotprod10/2
  dotprod1/1 -> Mux/1
  "IW{3,2}(2,:)'"/1 -> dotprod2/1
  dotprod2/1 -> Mux/2
  "IW{3,2}(3,:)'"/1 -> dotprod3/1
  dotprod3/1 -> Mux/3
  "IW{3,2}(4,:)'"/1 -> dotprod4/1
  dotprod4/1 -> Mux/4
  "IW{3,2}(5,:)'"/1 -> dotprod5/1
  dotprod5/1 -> Mux/5
  "IW{3,2}(6,:)'"/1 -> dotprod6/1
  dotprod6/1 -> Mux/6
  "IW{3,2}(7,:)'"/1 -> dotprod7/1
  dotprod7/1 -> Mux/7
  "IW{3,2}(8,:)'"/1 -> dotprod8/1
  dotprod8/1 -> Mux/8
  "IW{3,2}(9,:)'"/1 -> dotprod9/1
  dotprod9/1 -> Mux/9
  "IW{3,2}(10,:)'"/1 -> dotprod10/1
  dotprod10/1 -> Mux/10
  Mux/1 -> "lz{3,2}"/1

== system state_space_all_reduce_uio/Function Fitting Neural Network3/Layer 4/Delays 1 ==
  "p{4}" : Inport  PortDimensions=10  SampleTime=4e-05
      mask Display: e = 0.06;c1 = [120 230 180]/255;c2 = ([120 230 180]+0)/(256+128);c3 = ([120 230 180]+128)/(256+128);patch([0 1 1 0],[0 0 1 1],c1);patch([0 1 1 1-e 1-e 0+e],[0 0 1 1-e 0+e 0+e],c2);patch([0 0 1 1-e 0+e 0+e],[0 1 1 1-e 1-e 0+e],c3);plot([0 1 1 0 0],[0 0 1 1 0]);
  mux : Mux  Inputs=1
      mask Display: e = 0.06;c1 = [120 150 230]/255;c2 = ([120 150 230]+0)/383;c3 = ([120 150 230]+128)/383;patch([0 1 1 0],[0 0 1 1],c1);patch([0 1 1 1-e 1-e 0+e],[0 0 1 1-e 0+e 0+e],c2);patch([0 0 1 1-e 0+e 0+e],[0 1 1 1-e 1-e 0+e],c3);plot([0 1 1 0 0],[0 0 1 1 0]);disp('Mux')
  "pd{4,3}" : Outport
      mask Display: e = 0.06;c1 = [120 230 180]/255;c2 = ([120 230 180]+0)/(256+128);c3 = ([120 230 180]+128)/(256+128);patch([0 1 1 0],[0 0 1 1],c1);patch([0 1 1 1-e 1-e 0+e],[0 0 1 1-e 0+e 0+e],c2);patch([0 0 1 1-e 0+e 0+e],[0 1 1 1-e 1-e 0+e],c3);plot([0 1 1 0 0],[0 0 1 1 0]);
  wires:
  "p{4}"/1 -> mux/1
  mux/1 -> "pd{4,3}"/1

== system state_space_all_reduce_uio/Function Fitting Neural Network3/Layer 4/LW{4,3} ==
  "ad{4,3}" : Inport  PortDimensions=10  SampleTime=4e-05
      mask Display: e = 0.06;c1 = [120 230 180]/255;c2 = ([120 230 180]+0)/(256+128);c3 = ([120 230 180]+128)/(256+128);patch([0 1 1 0],[0 0 1 1],c1);patch([0 1 1 1-e 1-e 0+e],[0 0 1 1-e 0+e 0+e],c2);patch([0 0 1 1-e 0+e 0+e],[0 1 1 1-e 1-e 0+e],c3);plot([0 1 1 0 0],[0 0 1 1 0]);
  "IW{4,3}(1,:)'" : Constant  Value=[-0.91519999609158186881785468358430080115795135498046875;-0.64194219490654658155648348838440142571926116943359375;-0.658961222428368298409395720227621495723724365234375;0.190195201107200506651651039646822027862071990966796875;0.2000856511155351957764736425815499387681484222412109375;0.888469987290400720070238094194792211055755615234375;0.0032957608980333798730233407781042842543683946132659912109375;0.98687372165675413260288451056112535297870635986328125;-0.1442770203930148487092566256251302547752857208251953125;0.836578383821700466427273568115197122097015380859375]
      mask Display: e = 0.06;c1 = [120 150 230]/255;c2 = ([120 150 230]+0)/383;c3 = ([120 150 230]+128)/383;patch([0 1 1 0],[0 0 1 1],c1);patch([0 1 1 1-e 1-e 0+e],[0 0 1 1-e 0+e 0+e],c2);patch([0 0 1 1-e 0+e 0+e],[0 1 1 1-e 1-e 0+e],c3);plot([0 1 1 0 0],[0 0 1 1 0]);disp('weights');
  Mux : Mux  Inputs=1
      mask Display: e = 0.06;c1 = [120 150 230]/255;c2 = ([120 150 230]+0)/383;c3 = ([120 150 230]+128)/383;patch([0 1 1 0],[0 0 1 1],c1);patch([0 1 1 1-e 1-e 0+e],[0 0 1 1-e 0+e 0+e],c2);patch([0 0 1 1-e 0+e 0+e],[0 1 1 1-e 1-e 0+e],c3);plot([0 1 1 0 0],[0 0 1 1 0]);disp('Mux');
  dotprod1 : neural/Weight Functions/dotprod
  "lz{4,3}" : Outport
      mask Display: e = 0.06;c1 = [120 230 180]/255;c2 = ([120 230 180]+0)/(256+128);c3 = ([120 230 180]+128)/(256+128);patch([0 1 1 0],[0 0 1 1],c1);patch([0 1 1 1-e 1-e 0+e],[0 0 1 1-e 0+e 0+e],c2);patch([0 0 1 1-e 0+e 0+e],[0 1 1 1-e 1-e 0+e],c3);plot([0 1 1 0 0],[0 0 1 1 0]);
  wires:
  "IW{4,3}(1,:)'"/1 -> dotprod1/1
  "ad{4,3}"/1 -> dotprod1/2
  dotprod1/1 -> Mux/1
  Mux/1 -> "lz{4,3}"/1

== system state_space_all_reduce_uio/Function Fitting Neural Network4/Layer 1/Delays 1 ==
  "p{1}" : Inport  PortDimensions=44  SampleTime=4e-05
      mask Display: e = 0.06;c1 = [120 230 180]/255;c2 = ([120 230 180]+0)/(256+128);c3 = ([120 230 180]+128)/(256+128);patch([0 1 1 0],[0 0 1 1],c1);patch([0 1 1 1-e 1-e 0+e],[0 0 1 1-e 0+e 0+e],c2);patch([0 0 1 1-e 0+e 0+e],[0 1 1 1-e 1-e 0+e],c3);plot([0 1 1 0 0],[0 0 1 1 0]);
  mux : Mux  Inputs=1
      mask Display: e = 0.06;c1 = [120 150 230]/255;c2 = ([120 150 230]+0)/383;c3 = ([120 150 230]+128)/383;patch([0 1 1 0],[0 0 1 1],c1);patch([0 1 1 1-e 1-e 0+e],[0 0 1 1-e 0+e 0+e],c2);patch([0 0 1 1-e 0+e 0+e],[0 1 1 1-e 1-e 0+e],c3);plot([0 1 1 0 0],[0 0 1 1 0]);disp('Mux')
  "pd{1,1}" : Outport
      mask Display: e = 0.06;c1 = [120 230 180]/255;c2 = ([120 230 180]+0)/(256+128);c3 = ([120 230 180]+128)/(256+128);patch([0 1 1 0],[0 0 1 1],c1);patch([0 1 1 1-e 1-e 0+e],[0 0 1 1-e 0+e 0+e],c2);patch([0 0 1 1-e 0+e 0+e],[0 1 1 1-e 1-e 0+e],c3);plot([0 1 1 0 0],[0 0 1 1 0]);
  wires:
  "p{1}"/1 -> mux/1
  mux/1 -> "pd{1,1}"/1
